simulink library "csc_sim_simulation_lib"  (R2015b)
settings: Solver=ode45  StartTime=0.0  StopTime=10.0  RelTol=1e-3
values from neighbouring files (symbols this model uses):
  central_body_radius = gbl_param.earth_radius    [set_central_body_radius.m]
undefined symbols (not defined in the file or in its folder): central_body_flattening, central_body_rotation_rate, ini_alt_wrt_meanrad, ini_epoch_seconds, sim_time_step_size, swm_num_switches
libraries: util_common_lib x4, util_info_lib x1, util_frame_rotation_lib x1, telem_conversion_lib x1, csc_enf_environmental_forces_lib x1, csc_pwr_power_system_sim_lib x1, csc_rigid_body_dynamics_lib x1, csc_sensors_lib_a x1, csc_thl_thrusters_lander_lib x1, csu_isb_initialize_state_bus_lib x1, csu_mpl_mass_properties_lander_lib x1
settings Model: Creator=Mark Agbayani  LastModifiedBy=Mark Agbayani
settings DataIOCC: SaveFormat=Array
settings DebuggingCC: SolverPrmCheckMsg=warning
settings HardwareCC: ProdBitPerPointer=32  ProdLargestAtomicFloat=None  ProdIntDivRoundTo=Undefined  ProdEndianess=Unspecified  ProdWordSize=32  ProdHWDeviceType=32-bit Generic
settings GRTTargetCC: GeneratePreprocessorConditionals=Disable all
settings ConfigComp: CovModelRefEnable=Off  CovSFcnEnable=off

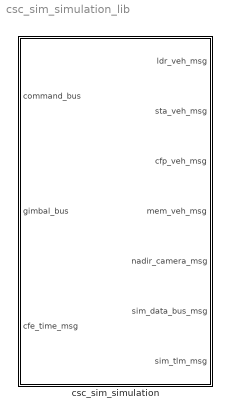
== system csc_sim_simulation_lib ==
  csc_sim_simulation : Subsystem  Tag=GSSE; MDL_TICK=THR_SIM_MSG  TreatAsAtomicUnit=on  SystemSampleTime=sim_time_step_size

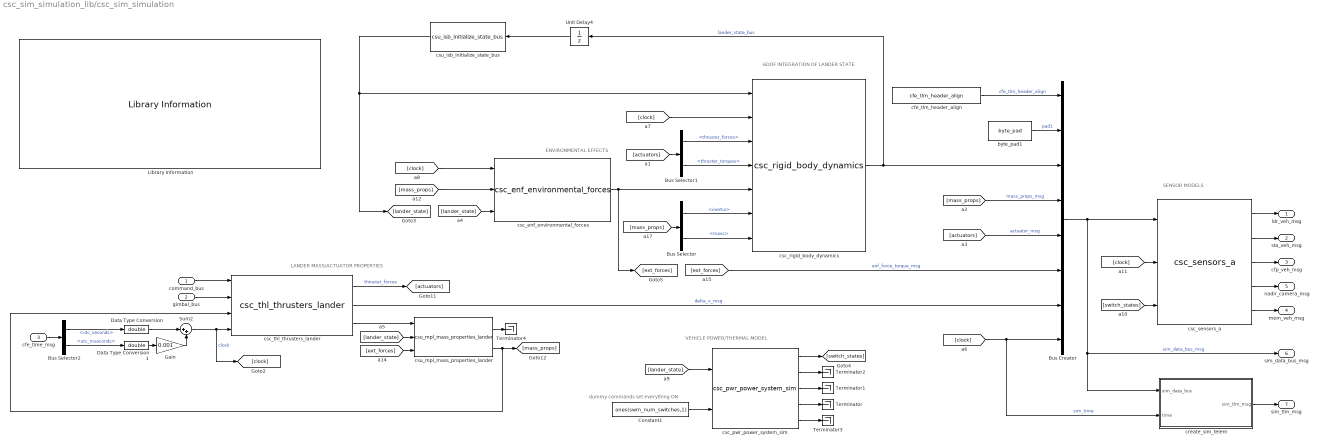
== system csc_sim_simulation_lib/csc_sim_simulation ==
  note: LANDER MASS/ACTUATOR PROPERTIES
  note: 6DOF INTEGRATION OF LANDER STATE
  note: ENVIRONMENTAL EFFECTS
  note: SENSOR MODELS
  note: VEHICLE POWER/THERMAL MODEL
  note: dummy commands set everything ON
  command_bus : Inport
  gimbal_bus : Inport  Port=2
  cfe_time_msg : Inport  Port=3  OutDataTypeStr=Bus: cfe_time_msg
  Bus Creator : BusCreator  Inputs=8  OutDataTypeStr=Bus: sim_data_bus_msg  NonVirtualBus=on
  Bus Selector : BusSelector  OutputSignals=inertia,mass
  Bus Selector1 : BusSelector  OutputSignals=thruster_forces,thruster_torques
  Bus Selector2 : BusSelector  OutputSignals=utc_seconds,utc_mseconds
  Constant1 : Constant  Value=ones(swm_num_switches,1)  OutDataTypeStr=double
  Data Type Conversion : DataTypeConversion  OutDataTypeStr=double
  Data Type Conversion1 : DataTypeConversion  OutDataTypeStr=double
  Gain : Gain  Gain=0.001
  Library Information : util_info_lib/Library Information  owner='NONE'
  Sum2 : Sum  Inputs=|++
  Terminator{,1..4} (5 alike) : Terminator
  Unit Delay4 : UnitDelay  SampleTime=-1
  byte_pad1 : util_common_lib/byte_pad  n_bytes=4
  cfe_tlm_header_align : util_common_lib/cfe_tlm_header_align
  create_sim_telem : Subsystem
  csc_enf_environmental_forces : csc_enf_environmental_forces_lib/csc_enf_environmental_forces
  csc_pwr_power_system_sim : csc_pwr_power_system_sim_lib/csc_pwr_power_system_sim
  csc_rigid_body_dynamics : csc_rigid_body_dynamics_lib/csc_rigid_body_dynamics
  csc_sensors_a : csc_sensors_lib_a/csc_sensors_a
  csc_thl_thrusters_lander : csc_thl_thrusters_lander_lib/csc_thl_thrusters_lander
  csu_isb_initialize_state_bus : csu_isb_initialize_state_bus_lib/csu_isb_initialize_state_bus
  csu_mpl_mass_properties_lander : csu_mpl_mass_properties_lander_lib/csu_mpl_mass_properties_lander
  ldr_veh_msg : Outport
  sta_veh_msg : Outport  Port=2
  cfp_veh_msg : Outport  Port=3
  mem_veh_msg : Outport  Port=4
  nadir_camera_msg : Outport  Port=5
  sim_data_bus_msg : Outport  Port=6
  sim_tlm_msg : Outport  Port=7
  wires:
  gimbal_bus/1 -> csc_thl_thrusters_lander/2
  cfe_time_msg/1 -> Bus Selector2/1
  Bus Selector2/2 -> Data Type Conversion1/1  "<utc_mseconds>"
  Data Type Conversion/1 -> Sum2/1
  Data Type Conversion1/1 -> Gain/1
  Gain/1 -> Sum2/2
  Bus Selector2/1 -> Data Type Conversion/1  "<utc_seconds>"
  byte_pad1/1 -> Bus Creator/2  "pad1"
  Sum2/1 -> [clock], csc_thl_thrusters_lander/4  "clock"
  [clock] -> create_sim_telem/2(time), Bus Creator/8  "sim_time"
  create_sim_telem/1(sim_tlm_msg) -> sim_tlm_msg/1
  Bus Creator/1 -> create_sim_telem/1(sim_data_bus), sim_data_bus_msg/1, csc_sensors_a/1  "sim_data_bus_msg"
  csc_rigid_body_dynamics/1 -> Bus Creator/3, Unit Delay4/1  "lander_state_bus"
  csc_sensors_a/3 -> cfp_veh_msg/1
  csc_sensors_a/4 -> nadir_camera_msg/1
  command_bus/1 -> csc_thl_thrusters_lander/1
  [actuators] -> Bus Creator/5  "actuator_msg"
  [mass_props] -> Bus Creator/4  "mass_props_msg"
  csu_mpl_mass_properties_lander/2 -> csc_thl_thrusters_lander/3, [mass_props]
  csc_sensors_a/2 -> sta_veh_msg/1
  csc_sensors_a/1 -> ldr_veh_msg/1
  csc_thl_thrusters_lander/3 -> csu_mpl_mass_properties_lander/1
  csc_thl_thrusters_lander/1 -> [actuators]  "thruster_forces"
  csc_thl_thrusters_lander/2 -> Bus Creator/7  "delta_v_msg"
  [clock] -> csc_enf_environmental_forces/1
  [mass_props] -> csc_enf_environmental_forces/2
  cfe_tlm_header_align/1 -> Bus Creator/1  "cfe_tlm_header_align"
  [clock] -> csc_rigid_body_dynamics/2
  [mass_props] -> Bus Selector/1
  Bus Selector/2 -> csc_rigid_body_dynamics/7  "<mass>"
  Bus Selector/1 -> csc_rigid_body_dynamics/6  "<inertia>"
  Bus Selector1/1 -> csc_rigid_body_dynamics/3  "<thruster_forces>"
  Bus Selector1/2 -> csc_rigid_body_dynamics/4  "<thruster_torques>"
  Unit Delay4/1 -> csu_isb_initialize_state_bus/1
  csu_isb_initialize_state_bus/1 -> csc_rigid_body_dynamics/1, [lander_state]
  [actuators] -> Bus Selector1/1
  csc_pwr_power_system_sim/4 -> Terminator/1
  csc_pwr_power_system_sim/3 -> Terminator1/1
  csc_pwr_power_system_sim/2 -> Terminator2/1
  csc_pwr_power_system_sim/1 -> [switch_states]
  [lander_state] -> csc_enf_environmental_forces/3
  [lander_state] -> csc_pwr_power_system_sim/1
  [clock] -> csc_sensors_a/2
  [switch_states] -> csc_sensors_a/3
  Constant1/1 -> csc_pwr_power_system_sim/2
  csc_sensors_a/5 -> mem_veh_msg/1
  csc_pwr_power_system_sim/5 -> Terminator3/1
  csu_mpl_mass_properties_lander/1 -> Terminator4/1
  [lander_state] -> csu_mpl_mass_properties_lander/2
  [ext_forces] -> csu_mpl_mass_properties_lander/3
  csc_enf_environmental_forces/1 -> [ext_forces], csc_rigid_body_dynamics/5
  [ext_forces] -> Bus Creator/6  "enf_force_torque_msg"

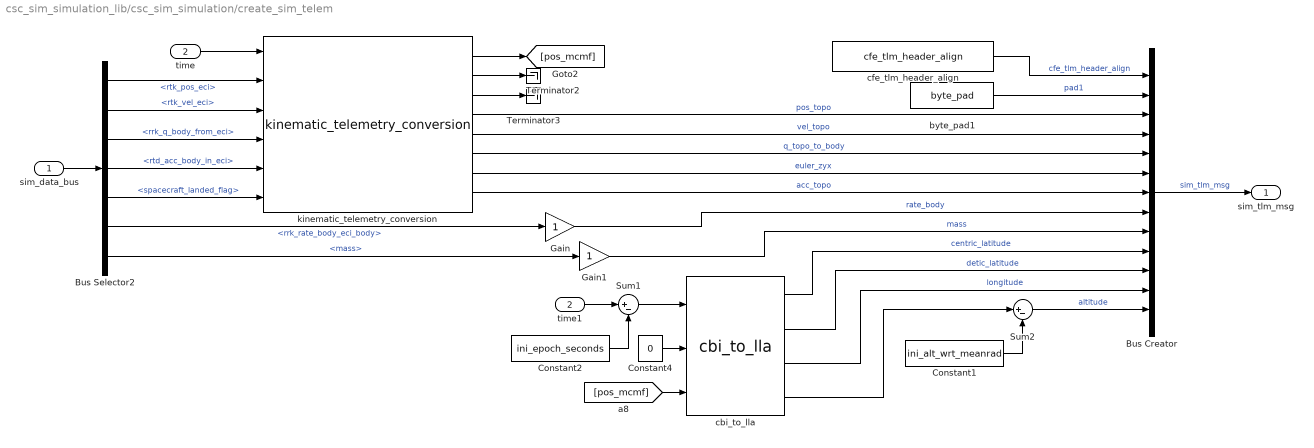
== system csc_sim_simulation_lib/csc_sim_simulation/create_sim_telem ==
  sim_data_bus : Inport
  time : Inport  Port=2
  Bus Creator : BusCreator  Inputs=13  OutDataTypeStr=Bus: sim_tlm_msg  NonVirtualBus=on
  Bus Selector2 : BusSelector  OutputSignals=lander_state_bus.rtk_pos_eci,lander_state_bus.rtk_vel_eci,lander_state_bus.rrk_q_body_from_eci,lander_state_bus.rtd_acc_body_in_eci,lander_state_bus.spacecraft_landed_flag,lander_state_bus.rrk_rate_body_eci_body,mass_props_msg.mass
  Constant1 : Constant  Value=ini_alt_wrt_meanrad  OutDataTypeStr=double
  Constant2 : Constant  Value=ini_epoch_seconds  OutDataTypeStr=double
  Constant4 : Constant  Value=0
  Gain : Gain
  Gain1 : Gain
  Sum1 : Sum  Inputs=|+-
  Sum2 : Sum  Inputs=|+-
  Terminator2 : Terminator
  Terminator3 : Terminator
  byte_pad1 : util_common_lib/byte_pad  n_bytes=4
  cbi_to_lla : util_frame_rotation_lib/cbi_to_lla  a=central_body_radius  b=central_body_radius*(1-central_body_flattening)  omega=central_body_rotation_rate(3)
  cfe_tlm_header_align : util_common_lib/cfe_tlm_header_align
  kinematic_telemetry_conversion : telem_conversion_lib/kinematic_telemetry_conversion
  time1 : InportShadow  Port=2
  sim_tlm_msg : Outport
  wires:
  Constant1/1 -> Sum2/2
  cbi_to_lla/4 -> Sum2/1
  kinematic_telemetry_conversion/1 -> [pos_mcmf]
  [pos_mcmf] -> cbi_to_lla/3
  Constant2/1 -> Sum1/2
  time1/1 -> Sum1/1
  Sum1/1 -> cbi_to_lla/1
  Constant4/1 -> cbi_to_lla/2
  Sum2/1 -> Bus Creator/13  "altitude"
  cbi_to_lla/3 -> Bus Creator/12  "longitude"
  cbi_to_lla/1 -> Bus Creator/10  "centric_latitude"
  cbi_to_lla/2 -> Bus Creator/11  "detic_latitude"
  Bus Selector2/5 -> kinematic_telemetry_conversion/6  "<spacecraft_landed_flag>"
  cfe_tlm_header_align/1 -> Bus Creator/1  "cfe_tlm_header_align"
  kinematic_telemetry_conversion/4 -> Bus Creator/3  "pos_topo"
  Gain1/1 -> Bus Creator/9  "mass"
  Bus Selector2/7 -> Gain1/1  "<mass>"
  Gain/1 -> Bus Creator/8  "rate_body"
  Bus Selector2/6 -> Gain/1  "<rrk_rate_body_eci_body>"
  Bus Selector2/4 -> kinematic_telemetry_conversion/5  "<rtd_acc_body_in_eci>"
  Bus Selector2/3 -> kinematic_telemetry_conversion/4  "<rrk_q_body_from_eci>"
  Bus Selector2/2 -> kinematic_telemetry_conversion/3  "<rtk_vel_eci>"
  Bus Selector2/1 -> kinematic_telemetry_conversion/2  "<rtk_pos_eci>"
  time/1 -> kinematic_telemetry_conversion/1
  sim_data_bus/1 -> Bus Selector2/1
  kinematic_telemetry_conversion/5 -> Bus Creator/4  "vel_topo"
  kinematic_telemetry_conversion/6 -> Bus Creator/5  "q_topo_to_body"
  kinematic_telemetry_conversion/7 -> Bus Creator/6  "euler_zyx"
  kinematic_telemetry_conversion/8 -> Bus Creator/7  "acc_topo"
  Bus Creator/1 -> sim_tlm_msg/1  "sim_tlm_msg"
  kinematic_telemetry_conversion/2 -> Terminator2/1
  kinematic_telemetry_conversion/3 -> Terminator3/1
  byte_pad1/1 -> Bus Creator/2  "pad1"
